simulink model "lab4_1Copy"  (R2020a)
settings: Solver=VariableStepAuto  StartTime=0.0  StopTime=20.0  RelTol=10e-10  AbsTol=10e-10
values from neighbouring files (symbols this model uses):
  d_bar = (Ra/Kt)*(tau_1)    (= 3)    [Lab4.m]    (also in lab4.m)
  thetades = pi/2    (= 1.57079632679)    [Lab4.m]    (also in lab4.m)
  Vlim = 5    [Lab4.m]    (also in lab4.m)
libraries: cstblocks x2
settings Model: Creator=Adam Cassie  LastModifiedBy=Adam Cassie

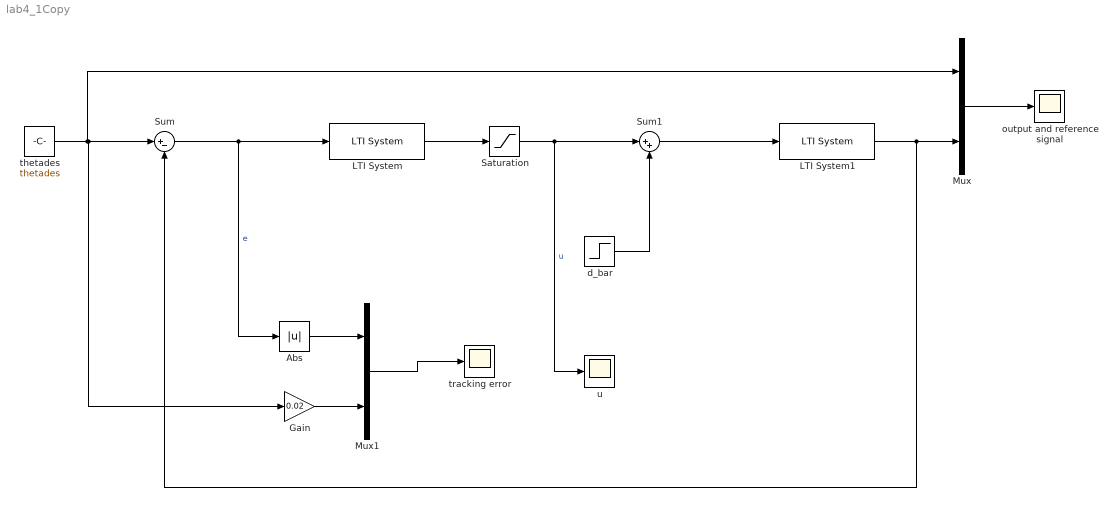
== system lab4_1Copy ==
  Abs : Abs
  Gain : Gain  Gain=0.02
  LTI System : cstblocks/LTI System  sys=C  IC=[]
  LTI System1 : cstblocks/LTI System  sys=G  IC=[]
  Mux : Mux  Inputs=2
  Mux1 : Mux  Inputs=2
  Saturation : Saturate  UpperLimit=Vlim  LowerLimit=-Vlim
  Sum : Sum  Inputs=|+-
  Sum1 : Sum  Inputs=|++
  d_bar : Step  Time=5  After=d_bar  SampleTime=0
  output and reference signal : Scope
  thetades : Constant  Value=thetades
  tracking error : Scope
  u : Scope
  wires:
  thetades/1 -> Gain/1, Sum/1, Mux/1
  Sum/1 -> Abs/1, LTI System/1  "e"
  LTI System/1 -> Saturation/1
  Sum1/1 -> LTI System1/1
  d_bar/1 -> Sum1/2
  LTI System1/1 -> Sum/2, Mux/2
  Mux/1 -> output and reference signal/1
  Saturation/1 -> u/1, Sum1/1  "u"
  Gain/1 -> Mux1/2
  Abs/1 -> Mux1/1
  Mux1/1 -> tracking error/1
